simulink model "SIM6"  (R2023b)
settings: Solver=ode4  StartTime=0.0  StopTime=tf  FixedStep=dt  RelTol=1e-3
InitFcn:
  | I = diag([3,4,2]);
  | % I = diag([60 39 42]);
  | % I = diag([2 3 4]);
  | Iinv = inv(I);
  | 
  | dt = 0.002;
  | dtsim = .1;
  | dtdata = 1;
  | dtcontrol = 0.08;
  | 
  | yaw0 = pi/4;
  | pitch0 = -pi/3;
  | roll0 = 3*pi/4;
  | 
  | % 3 2 1 sequence
  | DCM0 = [cos(yaw0) sin(yaw0) 0; -sin(yaw0) cos(yaw0) 0; 0 0 1]*...
  |       [cos(pitch0) 0 -sin(pitch0); 0 1 0; sin(pitch0) 0 cos(pitch0)]*...
  |       [1 0 0; 0 cos(roll0) sin(roll0); 0 -sin(roll0) cos(roll0)];
  | 
  | q4 = .5*sqrt(trace(DCM0)+1);
  | qhat = .25/q4*[DCM0(2,3) - DCM0(3,2); DCM0(3,1) - DCM0(1,3); DCM0(1,2) - DCM0(2,1)];
  | q0 = [qhat;q4];
  | w0 = [0;0;0];
  | qTarget = [0;0;0;1];
  | 
  | % order for gains is R-P-Y
  | Ki = diag([0,0,0]);
  | Kp = diag((0.11277)^2*[3,4,2]);
  | Kd = diag(2*.59115*(0.11277)*[3,4,2]);
  | 
  | 
  | mu = 398600; %km3/s2
  | H0 = [0;0;0];
  | r0 = [6678; 0; 0];
  | v0 = sqrt(mu/norm(r0))*[0;1; sqrt(3)]/2;
  | 
  | a = -mu/2/(norm(v0)^2/2 - mu/norm(r0));
  | % tf = 2*pi*sqrt(a^3/mu);
  | 
  | tf = 5*60;
  | 
  | myworld = vrworld('SpacecraftEarth.wrl');
  | 
  | open(myworld);
  | 
  | set(0,'Units','pixels');
  | 
  | scnsize = get(0,'ScreenSize');
  | 
  | vrsetpref DefaultFigurePlaneClipMethod bvolume
  | 
  | f1 = vrfigure(myworld,[1 80 scnsize(3)/2 scnsize(4)/2]);
  | 
  | set(f1,'Viewpoint','WorldView')
  | 
  | f2 = vrfigure(myworld,[scnsize(3)/2 80 scnsize(3)/2 scnsize(4)/2]);
  | 
  | set(f2,'Viewpoint','NadirView')
StopFcn:
  | angles = out.EulerAngles.Data;
  | time = out.EulerAngles.Time;
  | 
  | figure
  | subplot(1,3,1)
  | plot(time, angles(:,1), 'k');
  | ylabel("Yaw, rad")
  | xlabel("Time, s")
  | 
  | subplot(1,3,2)
  | plot(time, angles(:,2), 'k');
  | ylabel("Pitch, rad")
  | xlabel("Time, s")
  | 
  | subplot(1,3,3)
  | plot(time, angles(:,3), 'k');
  | ylabel("Roll, rad")
  | xlabel("Time, s")
undefined symbols (not defined in the file): DiscIntNeverNeededParam
libraries: vrlib x5, matrix_library x5
settings Model: Creator=David  LastModifiedBy=David

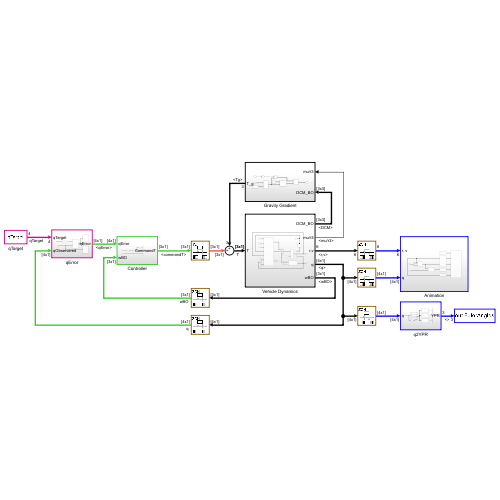
[thumbnail: Simulink's stored preview of the top-level diagram]
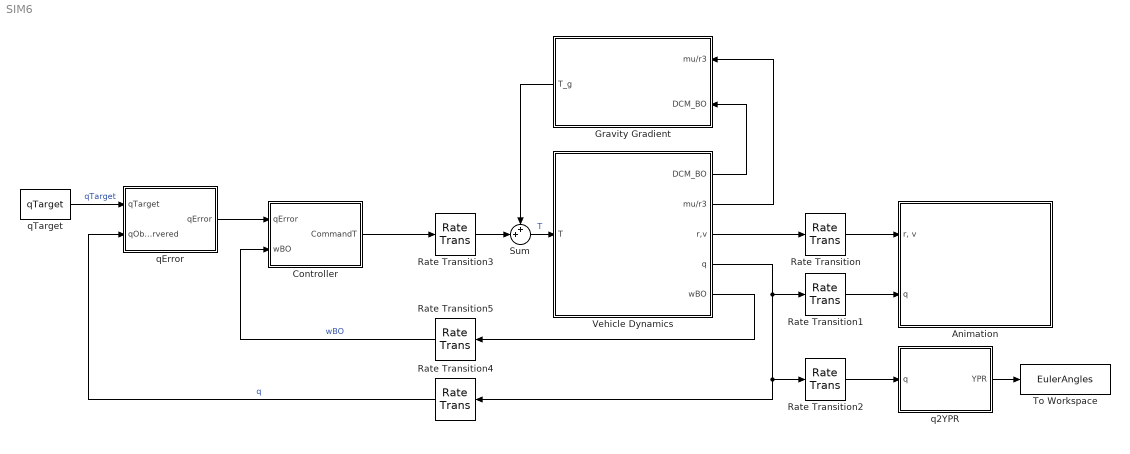
== system SIM6 ==
  Animation : Subsystem
  Controller : Subsystem
  Gravity Gradient : Subsystem
  Rate Transition : RateTransition  InitialCondition=[r0;v0]  OutPortSampleTime=dtsim
  Rate Transition1 : RateTransition  InitialCondition=q0  OutPortSampleTime=dtsim
  Rate Transition2 : RateTransition  InitialCondition=q0  OutPortSampleTime=dtdata
  Rate Transition3 : RateTransition  InitialCondition=[0;0;0]  OutPortSampleTime=dt
  Rate Transition4 : RateTransition  InitialCondition=q0  OutPortSampleTime=dtcontrol
  Rate Transition5 : RateTransition  InitialCondition=w0  OutPortSampleTime=dtcontrol
  Sum : Sum  Inputs=++|
  To Workspace : ToWorkspace  VariableName=EulerAngles  SaveFormat=Timeseries  SampleTime=-1
  Vehicle Dynamics : Subsystem
  q2YPR : Subsystem
  qError : Subsystem
  qTarget : Constant  Value=qTarget
  wires:
  Vehicle Dynamics/3(r,v) -> Rate Transition/1
  Vehicle Dynamics/4(q) -> Rate Transition2/1, Rate Transition4/1, Rate Transition1/1
  Rate Transition/1 -> Animation/1("r, v")
  Rate Transition1/1 -> Animation/2(q)
  Vehicle Dynamics/1(DCM_BO) -> Gravity Gradient/2(DCM_BO)
  Vehicle Dynamics/2(mu/r3) -> Gravity Gradient/1(mu/r3)
  q2YPR/1(YPR) -> To Workspace/1
  Rate Transition2/1 -> q2YPR/1(q)
  Sum/1 -> Vehicle Dynamics/1(T)  "T"
  Gravity Gradient/1(T_g) -> Sum/1
  Controller/1(CommandT) -> Rate Transition3/1
  Vehicle Dynamics/5(wBO) -> Rate Transition5/1
  Rate Transition3/1 -> Sum/2
  qError/1(qError) -> Controller/1(qError)
  qTarget/1 -> qError/1(qTarget)  "qTarget"
  Rate Transition4/1 -> qError/2(qObservered)  "q"
  Rate Transition5/1 -> Controller/2(wBO)  "wBO"

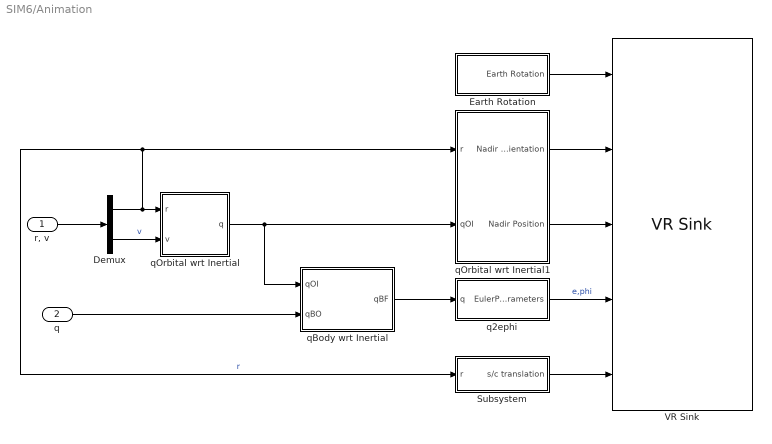
== system SIM6/Animation ==
  "r, v" : Inport
  q : Inport  Port=2
  Demux : Demux  Outputs=[3 3]
  Earth Rotation : Subsystem
  Subsystem : Subsystem
  VR Sink : vrlib/VR Sink  InstantiateOnLoad=on  SampleTime=dtsim  ViewEnable=on  RemoteChange=off  RemoteView=off  FieldsWritten=Earth.rotation.4.1.1.double#NadirView.orientation.4.1.1.double#NadirView.position.3.1.1.double#Spacecraft.rotation.4.1.1.double#Spacecraft.translation.3.1.1.double  WorldFileName=SpacecraftEarth.wrl  WorldDescription=The Earth - Low Resolution Model  AutoView=off  VideoDimensions=[]  AllowVariableSize=off
  q2ephi : Subsystem
  qBody wrt Inertial : Subsystem
  qOrbital wrt Inertial : Subsystem
  qOrbital wrt Inertial1 : Subsystem
  wires:
  "r, v"/1 -> Demux/1
  Demux/1 -> qOrbital wrt Inertial/1(r), Subsystem/1(r), qOrbital wrt Inertial1/1(r)  "r"
  Demux/2 -> qOrbital wrt Inertial/2(v)  "v"
  q/1 -> qBody wrt Inertial/2(qBO)
  qBody wrt Inertial/1(qBF) -> q2ephi/1(q)
  Earth Rotation/1(Earth Rotation) -> VR Sink/1
  q2ephi/1(EulerParameters) -> VR Sink/4  "e,phi"
  Subsystem/1(s/c translation) -> VR Sink/5
  qOrbital wrt Inertial1/1(Nadir Orientation) -> VR Sink/2
  qOrbital wrt Inertial1/2(Nadir Position) -> VR Sink/3
  qOrbital wrt Inertial/1(q) -> qBody wrt Inertial/1(qOI), qOrbital wrt Inertial1/2(qOI)

== system SIM6/Controller ==
  qError : Inport
  wBO : Inport  Port=2
  Discrete-Time Integrator : DiscreteIntegrator  SampleTime=dtcontrol  ICPrevOutput=DiscIntNeverNeededParam  ICPrevScaledInput=DiscIntNeverNeededParam
  Gain : Gain  Gain=2
  K : Gain  Gain=-[Ki, Kp, Kd]  Multiplication=Matrix(K*u)
  Mux : Mux  Inputs=3
  Selector : Selector  IndexOptions=Index vector (dialog)  Indices=1:3  OutputSizes=1
  CommandT : Outport  PortDimensions=[3,1]
  wires:
  qError/1 -> Selector/1
  Gain/1 -> Mux/2, Discrete-Time Integrator/1
  wBO/1 -> Mux/3
  Mux/1 -> K/1
  Selector/1 -> Gain/1  "thetaError"
  Discrete-Time Integrator/1 -> Mux/1
  K/1 -> CommandT/1  "commandT"

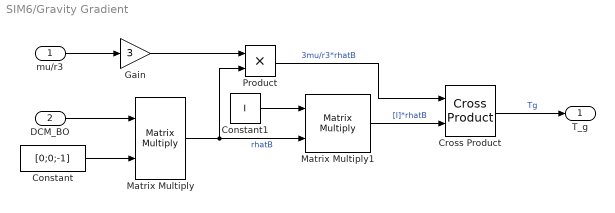
== system SIM6/Gravity Gradient ==
  mu/r3 : Inport
  DCM_BO : Inport  Port=2
  Constant : Constant  Value=[0;0;-1]
  Constant1 : Constant  Value=I
  Cross Product : matrix_library/Cross Product
  Gain : Gain  Gain=3
  Matrix Multiply : Product  Multiplication=Matrix(*)
  Matrix Multiply1 : Product  Multiplication=Matrix(*)
  Product : Product
  T_g : Outport
  wires:
  DCM_BO/1 -> Matrix Multiply/1
  Constant/1 -> Matrix Multiply/2
  mu/r3/1 -> Gain/1
  Matrix Multiply/1 -> Matrix Multiply1/2, Product/2  "rhatB"
  Matrix Multiply1/1 -> Cross Product/2  "[I]*rhatB"
  Gain/1 -> Product/1
  Product/1 -> Cross Product/1  "3mu/r3*rhatB"
  Cross Product/1 -> T_g/1  "Tg"
  Constant1/1 -> Matrix Multiply1/1

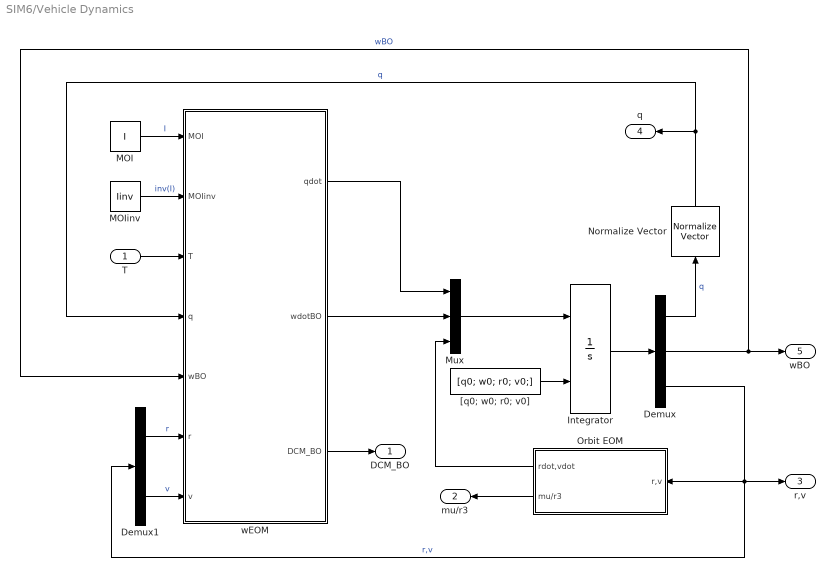
== system SIM6/Vehicle Dynamics ==
  T : Inport
  Demux : Demux  Outputs=[4, 3, 6]
  Demux1 : Demux  Outputs=2
  Integrator : Integrator  InitialConditionSource=external
  MOI : Constant  Value=I
  MOIinv : Constant  Value=Iinv
  Mux : Mux  Inputs=3
  Normalize Vector : vrlib/Utilities/Normalize Vector  maxzero=0
  Orbit EOM : Subsystem
  "[q0; w0; r0; v0]" : Constant  Value=[q0; w0; r0; v0;]
  wEOM : Subsystem
  DCM_BO : Outport
  mu/r3 : Outport  Port=2
  r,v : Outport  Port=3
  q : Outport  Port=4
  wBO : Outport  Port=5
  wires:
  MOI/1 -> wEOM/1(MOI)  "I"
  Integrator/1 -> Demux/1
  "[q0; w0; r0; v0]"/1 -> Integrator/2
  Normalize Vector/1 -> wEOM/4(q), q/1  "q"
  MOIinv/1 -> wEOM/2(MOIinv)  "inv(I)"
  Mux/1 -> Integrator/1
  Orbit EOM/1(rdot,vdot) -> Mux/3
  Demux/3 -> r,v/1, Demux1/1, Orbit EOM/1(r,v)  "r,v"
  Demux1/2 -> wEOM/7(v)  "v"
  Demux1/1 -> wEOM/6(r)  "r"
  Demux/2 -> wBO/1, wEOM/5(wBO)  "wBO"
  Demux/1 -> Normalize Vector/1  "q"
  wEOM/2(wdotBO) -> Mux/2
  wEOM/1(qdot) -> Mux/1
  T/1 -> wEOM/3(T)
  wEOM/3(DCM_BO) -> DCM_BO/1
  Orbit EOM/2(mu/r3) -> mu/r3/1

== system SIM6/q2YPR ==
  q : Inport  PortDimensions=[4,1]
  Bus Creator : BusCreator  Inputs=5
  Demux : Demux
  Mux : Mux  Inputs=3
  Square : Math  Operator=square
  q2theta1 : Subsystem
  q2theta2 : Subsystem
  q2theta3 : Subsystem
  YPR : Outport
  wires:
  q/1 -> Square/1, Demux/1
  Demux/1 -> Bus Creator/1  "q1"
  Demux/2 -> Bus Creator/2  "q2"
  Demux/3 -> Bus Creator/3  "q3"
  Demux/4 -> Bus Creator/4  "q4"
  Bus Creator/1 -> q2theta3/1(qBUS), q2theta1/1(qBUS), q2theta2/1(qBUS)
  q2theta1/1(Theta1) -> Mux/1  "theta1"
  q2theta2/1(Theta2) -> Mux/2  "theta2"
  q2theta3/1(Theta3) -> Mux/3  "theta3"
  Mux/1 -> YPR/1
  Square/1 -> Bus Creator/5  "q^2"

== system SIM6/qError ==
  qTarget : Inport
  qObservered : Inport  Port=2
  Display : Display
  Display1 : Display
  Gain : Gain  Gain=[-1;-1;-1;1]
  q*q' : Subsystem
  qError : Outport
  wires:
  q*q'/1(q'') -> Display/1, qError/1  "qError"
  qObservered/1 -> q*q'/2(q'), Display1/1  "q^-1"
  Gain/1 -> q*q'/1(q)  "q^-1"
  qTarget/1 -> Gain/1

== system SIM6/Animation/Earth Rotation ==
  Constant : Constant  Value=[0 0 1]
  Digital Clock : DigitalClock  SampleTime=dtsim
  Gain : Gain  Gain=2*pi/3600/24
  Mux : Mux  Inputs=2
  Earth Rotation : Outport
  wires:
  Digital Clock/1 -> Gain/1
  Gain/1 -> Mux/2  "phi"
  Mux/1 -> Earth Rotation/1  "e,phi"
  Constant/1 -> Mux/1  "e"

== system SIM6/Animation/Subsystem ==
  r : Inport
  Gain : Gain  Gain=1/6378
  s/c translation : Outport
  wires:
  r/1 -> Gain/1
  Gain/1 -> s/c translation/1  "r"

== system SIM6/Animation/q2ephi ==
  q : Inport  PortDimensions=[4;1]
  Acos : Trigonometry  Operator=acos
  Demux : Demux  Outputs=[3,1]
  Divide : Product  Inputs=*/
  Gain : Gain  Gain=2
  Mux : Mux  Inputs=2
  Sin : Trigonometry
  EulerParameters : Outport
  wires:
  q/1 -> Demux/1
  Acos/1 -> Gain/1, Sin/1  "phi/2"
  Sin/1 -> Divide/2
  Demux/1 -> Divide/1  "qhat"
  Demux/2 -> Acos/1  "q4"
  Divide/1 -> Mux/1  "e"
  Gain/1 -> Mux/2  "phi"
  Mux/1 -> EulerParameters/1

== system SIM6/Animation/qBody wrt Inertial ==
  qOI : Inport  PortDimensions=[4,1]
  qBO : Inport  Port=2  PortDimensions=[4,1]
  Demux : Demux
  Gain : Gain  Gain=[0,0,0,1;0,0,1,0;0,-1,0,0;-1,0,0,0]
  Gain1 : Gain  Gain=[0,0,-1,0;0,0,0,1;1,0,0,0;0,-1,0,0]
  Gain2 : Gain  Gain=[0,1,0,0;-1,0,0,0;0,0,0,1;0,0,-1,0]
  Gain3 : Gain  Gain=[1,0,0,0;0,1,0,0;0,0,1,0;0,0,0,1]
  Matrix Multiply : Product  Multiplication=Matrix(*)
  Sum : Sum  Inputs=++++
  qBF : Outport
  wires:
  Matrix Multiply/1 -> qBF/1  "qBF"
  qOI/1 -> Matrix Multiply/2
  Sum/1 -> Matrix Multiply/1
  Gain/1 -> Sum/1
  Gain1/1 -> Sum/2
  Gain3/1 -> Sum/4
  Gain2/1 -> Sum/3
  Demux/3 -> Gain2/1  "q3"
  Demux/4 -> Gain3/1  "q4"
  Demux/2 -> Gain1/1  "q2"
  Demux/1 -> Gain/1  "q1"
  qBO/1 -> Demux/1

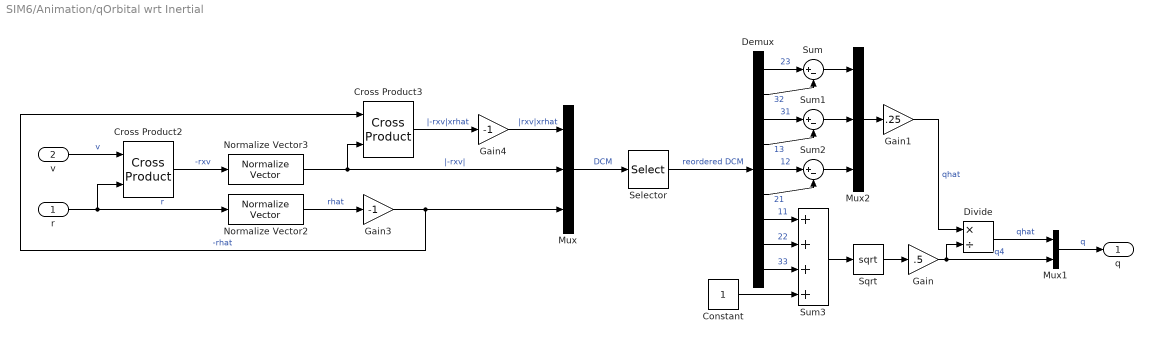
== system SIM6/Animation/qOrbital wrt Inertial ==
  r : Inport
  v : Inport  Port=2
  Constant : Constant
  Cross Product2 : matrix_library/Cross Product
  Cross Product3 : matrix_library/Cross Product
  Demux : Demux  Outputs=9
  Divide : Product  Inputs=*/
  Gain : Gain  Gain=.5
  Gain1 : Gain  Gain=.25
  Gain3 : Gain  Gain=-1
  Gain4 : Gain  Gain=-1
  Mux : Mux  Inputs=3
  Mux1 : Mux  Inputs=2
  Mux2 : Mux  Inputs=3
  Normalize Vector2 : vrlib/Utilities/Normalize Vector  maxzero=0
  Normalize Vector3 : vrlib/Utilities/Normalize Vector  maxzero=0
  Selector : Selector  InputPortWidth=9  IndexOptions=Index vector (dialog)  Indices=[6 8 7 3 2 4 1 5 9]  OutputSizes=1
  Sqrt : Sqrt
  Sum : Sum  Inputs=|+-
  Sum1 : Sum  Inputs=|+-
  Sum2 : Sum  Inputs=|+-
  Sum3 : Sum  Inputs=++++
  q : Outport
  wires:
  r/1 -> Cross Product2/2, Normalize Vector2/1  "r"
  Normalize Vector2/1 -> Gain3/1  "rhat"
  Gain3/1 -> Mux/3, Cross Product3/1  "-rhat"
  v/1 -> Cross Product2/1  "v"
  Normalize Vector3/1 -> Cross Product3/2, Mux/2  "|-rxv|"
  Cross Product2/1 -> Normalize Vector3/1  "-rxv"
  Cross Product3/1 -> Gain4/1  "|-rxv|xrhat"
  Gain4/1 -> Mux/1  "|rxv|xrhat"
  Mux1/1 -> q/1  "q"
  Divide/1 -> Mux1/1  "qhat"
  Gain/1 -> Mux1/2, Divide/2  "q4"
  Gain1/1 -> Divide/1  "qhat"
  Mux2/1 -> Gain1/1
  Sum2/1 -> Mux2/3
  Sum1/1 -> Mux2/2
  Sum/1 -> Mux2/1
  Sqrt/1 -> Gain/1
  Sum3/1 -> Sqrt/1
  Constant/1 -> Sum3/4
  Demux/9 -> Sum3/3  "33"
  Demux/7 -> Sum3/1  "11"
  Demux/6 -> Sum2/2  "21"
  Demux/5 -> Sum2/1  "12"
  Demux/2 -> Sum/2  "32"
  Demux/4 -> Sum1/2  "13"
  Demux/8 -> Sum3/2  "22"
  Demux/3 -> Sum1/1  "31"
  Demux/1 -> Sum/1  "23"
  Selector/1 -> Demux/1  "reordered DCM"
  Mux/1 -> Selector/1  "DCM"

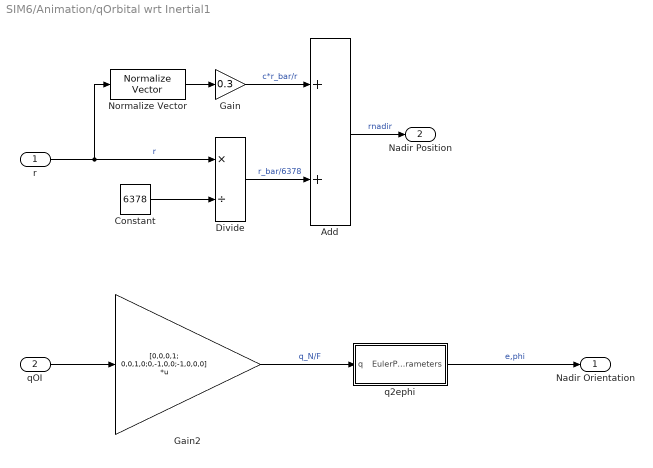
== system SIM6/Animation/qOrbital wrt Inertial1 ==
  r : Inport
  qOI : Inport  Port=2
  Add : Sum
  Constant : Constant  Value=6378
  Divide : Product  Inputs=*/
  Gain : Gain  Gain=0.3
  Gain2 : Gain  Gain=[0,0,0,1; 0,0,1,0;0,-1,0,0;-1,0,0,0]  Multiplication=Matrix(K*u)
  Normalize Vector : vrlib/Utilities/Normalize Vector  maxzero=0
  q2ephi : Subsystem
  Nadir Orientation : Outport
  Nadir Position : Outport  Port=2
  wires:
  qOI/1 -> Gain2/1
  Gain2/1 -> q2ephi/1(q)  "q_N/F"
  q2ephi/1(EulerParameters) -> Nadir Orientation/1  "e,phi"
  r/1 -> Normalize Vector/1, Divide/1  "r"
  Constant/1 -> Divide/2
  Divide/1 -> Add/2  "r_bar/6378"
  Add/1 -> Nadir Position/1  "rnadir"
  Normalize Vector/1 -> Gain/1
  Gain/1 -> Add/1  "c*r_bar/r"

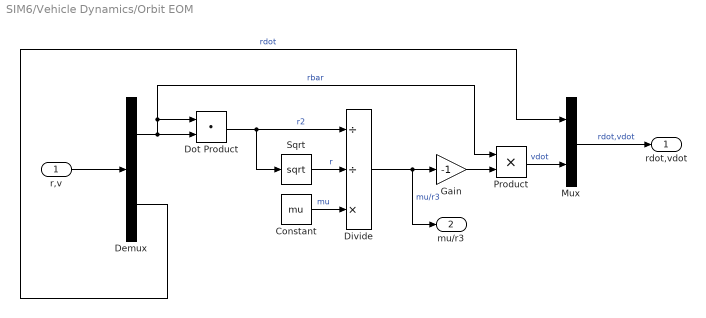
== system SIM6/Vehicle Dynamics/Orbit EOM ==
  r,v : Inport
  Constant : Constant  Value=mu
  Demux : Demux  Outputs=2
  Divide : Product  Inputs=//*
  Dot Product : DotProduct  OutDataTypeStr=Inherit: Inherit via internal rule
  Gain : Gain  Gain=-1
  Mux : Mux  Inputs=2
  Product : Product
  Sqrt : Sqrt
  rdot,vdot : Outport
  mu/r3 : Outport  Port=2
  wires:
  Demux/2 -> Mux/1  "rdot"
  Demux/1 -> Product/1, Dot Product/1, Dot Product/2  "rbar"
  Mux/1 -> rdot,vdot/1  "rdot,vdot"
  Divide/1 -> Gain/1, mu/r3/1  "mu/r3"
  r,v/1 -> Demux/1
  Dot Product/1 -> Divide/1, Sqrt/1  "r2"
  Constant/1 -> Divide/3  "mu"
  Sqrt/1 -> Divide/2  "r"
  Gain/1 -> Product/2
  Product/1 -> Mux/2  "vdot"

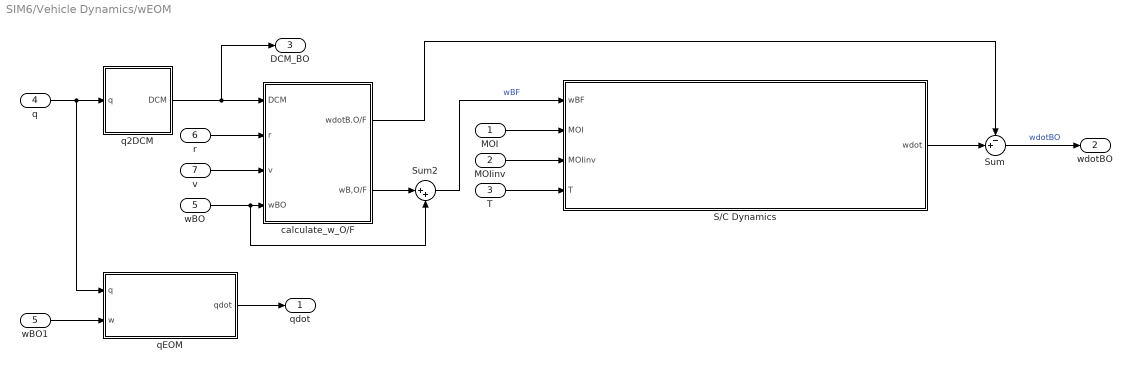
== system SIM6/Vehicle Dynamics/wEOM ==
  MOI : Inport
  MOIinv : Inport  Port=2
  T : Inport  Port=3
  q : Inport  Port=4
  wBO : Inport  Port=5
  r : Inport  Port=6
  v : Inport  Port=7
  S/C Dynamics : Subsystem
  Sum : Sum  Inputs=-+|
  Sum2 : Sum  Inputs=|++
  calculate_w_O/F : Subsystem
  q2DCM : Subsystem
  qEOM : Subsystem
  wBO1 : InportShadow  Port=5
  qdot : Outport
  wdotBO : Outport  Port=2
  DCM_BO : Outport  Port=3
  wires:
  q/1 -> qEOM/1(q), q2DCM/1(q)
  q2DCM/1(DCM) -> DCM_BO/1, calculate_w_O/F/1(DCM)
  r/1 -> calculate_w_O/F/2(r)
  v/1 -> calculate_w_O/F/3(v)
  wBO/1 -> Sum2/2, calculate_w_O/F/4(wBO)
  calculate_w_O/F/2(wB,O/F) -> Sum2/1
  S/C Dynamics/1(wdot) -> Sum/2
  calculate_w_O/F/1(wdotB.O/F) -> Sum/1
  T/1 -> S/C Dynamics/4(T)
  Sum/1 -> wdotBO/1  "wdotBO"
  Sum2/1 -> S/C Dynamics/1(wBF)  "wBF"
  MOI/1 -> S/C Dynamics/2(MOI)
  MOIinv/1 -> S/C Dynamics/3(MOIinv)
  wBO1/1 -> qEOM/2(w)
  qEOM/1(qdot) -> qdot/1

== system SIM6/q2YPR/q2theta1 ==
  qBUS : Inport
  Atan2 : Trigonometry  Operator=atan2
  Bus Selector : BusSelector  OutputSignals=q1,q2,q3,q4,q^2
  Demux : Demux
  Gain : Gain  Gain=2
  Product : Product
  Product1 : Product
  Sum : Sum  Inputs=|++
  Sum1 : Sum  Inputs=+--+
  Theta1 : Outport
  wires:
  qBUS/1 -> Bus Selector/1
  Atan2/1 -> Theta1/1
  Bus Selector/1 -> Product/1  "<q1>"
  Bus Selector/2 -> Product/2  "<q2>"
  Bus Selector/3 -> Product1/1  "<q3>"
  Bus Selector/4 -> Product1/2  "<q4>"
  Product/1 -> Sum/1
  Product1/1 -> Sum/2
  Sum/1 -> Gain/1
  Gain/1 -> Atan2/1
  Demux/1 -> Sum1/1
  Demux/2 -> Sum1/2
  Demux/3 -> Sum1/3
  Demux/4 -> Sum1/4
  Sum1/1 -> Atan2/2
  Bus Selector/5 -> Demux/1  "<q^2>"

== system SIM6/q2YPR/q2theta2 ==
  qBUS : Inport
  Asin : Trigonometry  Operator=asin
  Bus Selector : BusSelector  OutputSignals=q1,q3,q2,q4
  Gain : Gain  Gain=-2
  Product : Product
  Product1 : Product
  Subtract : Sum  Inputs=+-
  Theta2 : Outport
  wires:
  qBUS/1 -> Bus Selector/1
  Bus Selector/1 -> Product/1  "<q1>"
  Bus Selector/2 -> Product/2  "<q3>"
  Bus Selector/3 -> Product1/1  "<q2>"
  Bus Selector/4 -> Product1/2  "<q4>"
  Product/1 -> Subtract/1  "q1q3"
  Product1/1 -> Subtract/2  "q2q4"
  Subtract/1 -> Gain/1
  Gain/1 -> Asin/1
  Asin/1 -> Theta2/1

== system SIM6/q2YPR/q2theta3 ==
  qBUS : Inport
  Atan2 : Trigonometry  Operator=atan2
  Bus Selector : BusSelector  OutputSignals=q2,q3,q1,q4,q^2
  Demux : Demux
  Gain : Gain  Gain=2
  Product : Product
  Product1 : Product
  Sum : Sum  Inputs=|++
  Sum1 : Sum  Inputs=--++
  Theta3 : Outport
  wires:
  qBUS/1 -> Bus Selector/1
  Atan2/1 -> Theta3/1
  Product/1 -> Sum/1
  Product1/1 -> Sum/2
  Sum/1 -> Gain/1
  Gain/1 -> Atan2/1
  Demux/1 -> Sum1/1
  Demux/2 -> Sum1/2
  Demux/3 -> Sum1/3
  Demux/4 -> Sum1/4
  Sum1/1 -> Atan2/2
  Bus Selector/1 -> Product/1  "<q2>"
  Bus Selector/2 -> Product/2  "<q3>"
  Bus Selector/3 -> Product1/1  "<q1>"
  Bus Selector/4 -> Product1/2  "<q4>"
  Bus Selector/5 -> Demux/1  "<q^2>"

== system SIM6/qError/q*q' ==
  q : Inport  PortDimensions=[4,1]
  q' : Inport  Port=2  PortDimensions=[4,1]
  Demux : Demux
  Gain : Gain  Gain=[0,0,0,1;0,0,1,0;0,-1,0,0;-1,0,0,0]
  Gain1 : Gain  Gain=[0,0,-1,0;0,0,0,1;1,0,0,0;0,-1,0,0]
  Gain2 : Gain  Gain=[0,1,0,0;-1,0,0,0;0,0,0,1;0,0,-1,0]
  Gain3 : Gain  Gain=[1,0,0,0;0,1,0,0;0,0,1,0;0,0,0,1]
  Matrix Multiply : Product  Multiplication=Matrix(*)
  Sum : Sum  Inputs=++++
  q'' : Outport
  wires:
  q'/1 -> Demux/1
  Demux/1 -> Gain/1
  Demux/2 -> Gain1/1
  Demux/4 -> Gain3/1
  Demux/3 -> Gain2/1
  Gain2/1 -> Sum/3
  Gain3/1 -> Sum/4
  Gain1/1 -> Sum/2
  Gain/1 -> Sum/1
  Sum/1 -> Matrix Multiply/1
  q/1 -> Matrix Multiply/2
  Matrix Multiply/1 -> q''/1

== system SIM6/Animation/qOrbital wrt Inertial1/q2ephi ==
  q : Inport  PortDimensions=[4;1]
  Acos : Trigonometry  Operator=acos
  Demux : Demux  Outputs=[3,1]
  Divide : Product  Inputs=*/
  Gain : Gain  Gain=2
  Mux : Mux  Inputs=2
  Sin : Trigonometry
  EulerParameters : Outport
  wires:
  q/1 -> Demux/1
  Acos/1 -> Gain/1, Sin/1  "phi/2"
  Sin/1 -> Divide/2
  Demux/1 -> Divide/1  "qhat"
  Demux/2 -> Acos/1  "q4"
  Divide/1 -> Mux/1  "e"
  Gain/1 -> Mux/2  "phi"
  Mux/1 -> EulerParameters/1

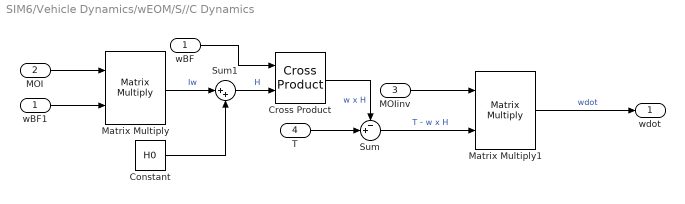
== system SIM6/Vehicle Dynamics/wEOM/S//C Dynamics ==
  wBF : Inport
  MOI : Inport  Port=2
  MOIinv : Inport  Port=3
  T : Inport  Port=4
  Constant : Constant  Value=H0
  Cross Product : matrix_library/Cross Product
  Matrix Multiply : Product  Multiplication=Matrix(*)
  Matrix Multiply1 : Product  Multiplication=Matrix(*)
  Sum : Sum  Inputs=-+|
  Sum1 : Sum  Inputs=|++
  wBF1 : InportShadow
  wdot : Outport
  wires:
  T/1 -> Sum/2
  Sum/1 -> Matrix Multiply1/2  "T - w x H"
  Cross Product/1 -> Sum/1  "w x H"
  MOIinv/1 -> Matrix Multiply1/1
  Constant/1 -> Sum1/2
  wBF/1 -> Cross Product/1
  Sum1/1 -> Cross Product/2  "H"
  Matrix Multiply/1 -> Sum1/1  "Iw"
  wBF1/1 -> Matrix Multiply/2
  MOI/1 -> Matrix Multiply/1
  Matrix Multiply1/1 -> wdot/1  "wdot"

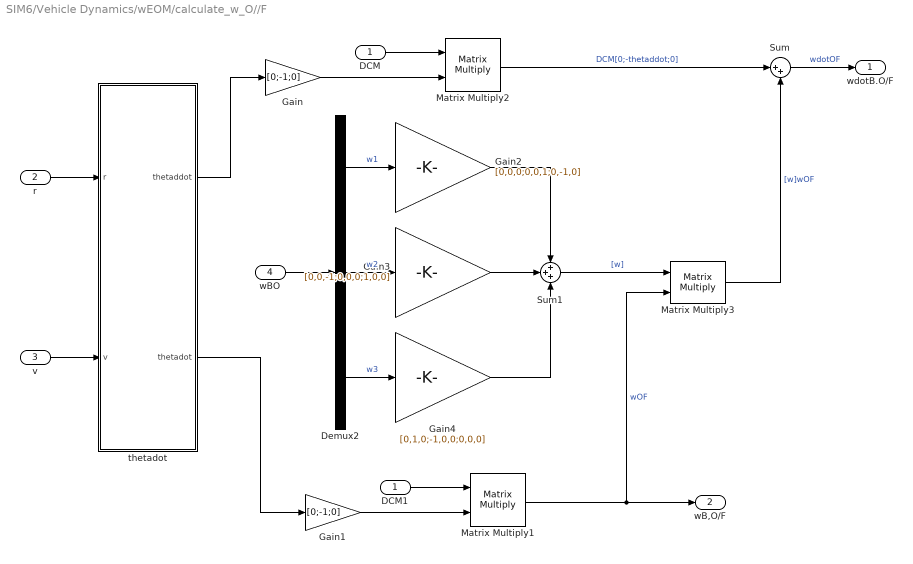
== system SIM6/Vehicle Dynamics/wEOM/calculate_w_O//F ==
  DCM : Inport
  r : Inport  Port=2
  v : Inport  Port=3
  wBO : Inport  Port=4
  DCM1 : InportShadow
  Demux2 : Demux  Outputs=3
  Gain : Gain  Gain=[0;-1;0]
  Gain1 : Gain  Gain=[0;-1;0]
  Gain2 : Gain  Gain=[0,0,0;0,0,1;0,-1,0]
  Gain3 : Gain  Gain=[0,0,-1;0,0,0;1,0,0]
  Gain4 : Gain  Gain=[0,1,0;-1,0,0;0,0,0]
  Matrix Multiply1 : Product  Multiplication=Matrix(*)
  Matrix Multiply2 : Product  Multiplication=Matrix(*)
  Matrix Multiply3 : Product  Multiplication=Matrix(*)
  Sum : Sum  Inputs=|++
  Sum1 : Sum  Inputs=+++
  thetadot : Subsystem
  wdotB.O/F : Outport
  wB,O/F : Outport  Port=2
  wires:
  r/1 -> thetadot/1(r)
  Gain/1 -> Matrix Multiply2/2
  v/1 -> thetadot/2(v)
  DCM/1 -> Matrix Multiply2/1
  Gain1/1 -> Matrix Multiply1/2
  Matrix Multiply1/1 -> Matrix Multiply3/2, wB,O/F/1  "wOF"
  DCM1/1 -> Matrix Multiply1/1
  Demux2/1 -> Gain2/1  "w1"
  wBO/1 -> Demux2/1
  Demux2/2 -> Gain3/1  "w2"
  Gain4/1 -> Sum1/3
  Gain3/1 -> Sum1/2
  Gain2/1 -> Sum1/1
  Matrix Multiply2/1 -> Sum/1  "DCM[0;-thetaddot;0]"
  Sum/1 -> wdotB.O/F/1  "wdotOF"
  thetadot/1(thetaddot) -> Gain/1
  thetadot/2(thetadot) -> Gain1/1
  Demux2/3 -> Gain4/1  "w3"
  Matrix Multiply3/1 -> Sum/2  "[w]wOF"
  Sum1/1 -> Matrix Multiply3/1  "[w]"

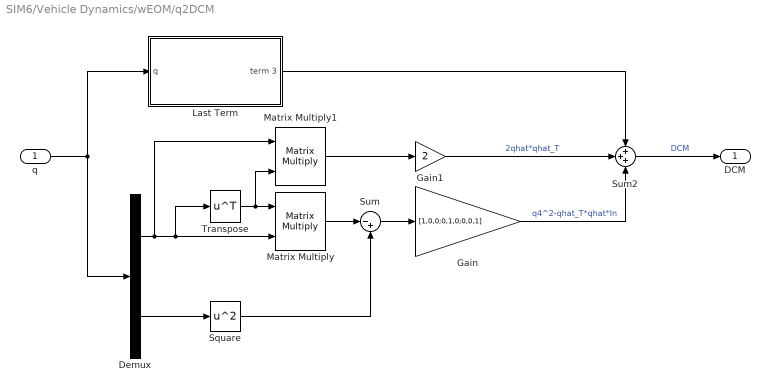
== system SIM6/Vehicle Dynamics/wEOM/q2DCM ==
  q : Inport  PortDimensions=[4,1]
  Demux : Demux  Outputs=[3,1]
  Gain : Gain  Gain=[1,0,0;0,1,0;0,0,1]
  Gain1 : Gain  Gain=2
  Last Term : Subsystem
  Matrix Multiply : Product  Multiplication=Matrix(*)
  Matrix Multiply1 : Product  Multiplication=Matrix(*)
  Square : Math  Operator=square
  Sum : Sum  Inputs=|-+
  Sum2 : Sum  Inputs=+++
  Transpose : Math  Operator=transpose
  DCM : Outport
  wires:
  Demux/2 -> Square/1
  Demux/1 -> Matrix Multiply1/1, Transpose/1, Matrix Multiply/2
  Transpose/1 -> Matrix Multiply1/2, Matrix Multiply/1
  Matrix Multiply/1 -> Sum/1
  Square/1 -> Sum/2
  Sum/1 -> Gain/1
  q/1 -> Last Term/1(q), Demux/1
  Matrix Multiply1/1 -> Gain1/1
  Sum2/1 -> DCM/1  "DCM"
  Last Term/1(term 3) -> Sum2/1
  Gain1/1 -> Sum2/2  "2qhat*qhat_T"
  Gain/1 -> Sum2/3  "q4^2-qhat_T*qhat*In"

== system SIM6/Vehicle Dynamics/wEOM/qEOM ==
  q : Inport
  w : Inport  Port=2
  Demux : Demux  Outputs=3
  Gain : Gain  Gain=.5
  Gain1 : Gain  Gain=[0,0,0,1;0,0,1,0;0,-1,0,0;-1,0,0,0]
  Gain2 : Gain  Gain=[0,0,-1,0;0,0,0,1;1,0,0,0;0,-1,0,0]
  Gain3 : Gain  Gain=[0,1,0,0;-1,0,0,0;0,0,0,1;0,0,-1,0]
  Matrix Multiply : Product  Multiplication=Matrix(*)
  Sum : Sum  Inputs=+++
  qdot : Outport
  wires:
  q/1 -> Gain/1
  Matrix Multiply/1 -> qdot/1  "qdot"
  Gain/1 -> Matrix Multiply/2  ".5 q"
  w/1 -> Demux/1
  Demux/1 -> Gain1/1  "w1"
  Demux/2 -> Gain2/1  "w2"
  Demux/3 -> Gain3/1  "w3"
  Gain2/1 -> Sum/2
  Gain3/1 -> Sum/3
  Gain1/1 -> Sum/1
  Sum/1 -> Matrix Multiply/1  "Omega"

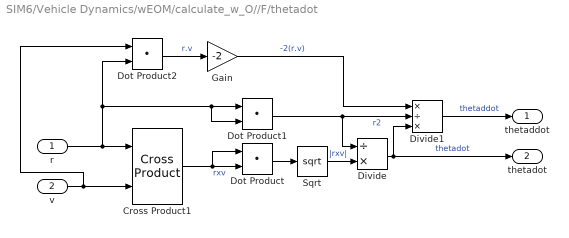
== system SIM6/Vehicle Dynamics/wEOM/calculate_w_O//F/thetadot ==
  r : Inport
  v : Inport  Port=2
  Cross Product1 : matrix_library/Cross Product
  Divide : Product  Inputs=/*
  Divide1 : Product  Inputs=*/*
  Dot Product : DotProduct  OutDataTypeStr=Inherit: Inherit via internal rule
  Dot Product1 : DotProduct  OutDataTypeStr=Inherit: Inherit via internal rule
  Dot Product2 : DotProduct  OutDataTypeStr=Inherit: Inherit via internal rule
  Gain : Gain  Gain=-2
  Sqrt : Sqrt
  thetaddot : Outport
  thetadot : Outport  Port=2
  wires:
  r/1 -> Dot Product1/1, Dot Product1/2, Dot Product2/2, Cross Product1/1
  Dot Product1/1 -> Divide1/2, Divide/1  "r2"
  Cross Product1/1 -> Dot Product/2, Dot Product/1  "rxv"
  v/1 -> Cross Product1/2, Dot Product2/1
  Sqrt/1 -> Divide/2  "|rxv|"
  Divide/1 -> thetadot/1, Divide1/3  "thetadot"
  Dot Product/1 -> Sqrt/1
  Dot Product2/1 -> Gain/1  "r.v"
  Gain/1 -> Divide1/1  "-2(r.v)"
  Divide1/1 -> thetaddot/1  "thetaddot"

== system SIM6/Vehicle Dynamics/wEOM/q2DCM/Last Term ==
  q : Inport
  Demux1 : Demux  Outputs=[3,1]
  Demux2 : Demux  Outputs=3
  Gain2 : Gain  Gain=[0,0,0;0,0,1;0,-1,0]
  Gain3 : Gain  Gain=[0,0,-1;0,0,0;1,0,0]
  Gain4 : Gain  Gain=[0,1,0;-1,0,0;0,0,0]
  Gain5 : Gain  Gain=2
  Product : Product
  Sum1 : Sum  Inputs=+++
  term 3 : Outport
  wires:
  Gain4/1 -> Sum1/3
  Demux2/3 -> Gain4/1
  Demux2/2 -> Gain3/1
  Demux1/2 -> Gain5/1
  Sum1/1 -> Product/1
  Gain2/1 -> Sum1/1
  Demux2/1 -> Gain2/1
  Gain3/1 -> Sum1/2
  Gain5/1 -> Product/2
  Demux1/1 -> Demux2/1
  Product/1 -> term 3/1
  q/1 -> Demux1/1
